simulink model "fuzzy_control_t2"  (R2017a)
settings: Solver=FixedStepAuto  StartTime=0.0  StopTime=10.0  FixedStep=0.0001  MaxStep=0.001  RelTol=1e-3
libraries: fuzblock x2
settings Model: Creator=Chaohua Zhao  LastModifiedBy=Chaohua Zhao

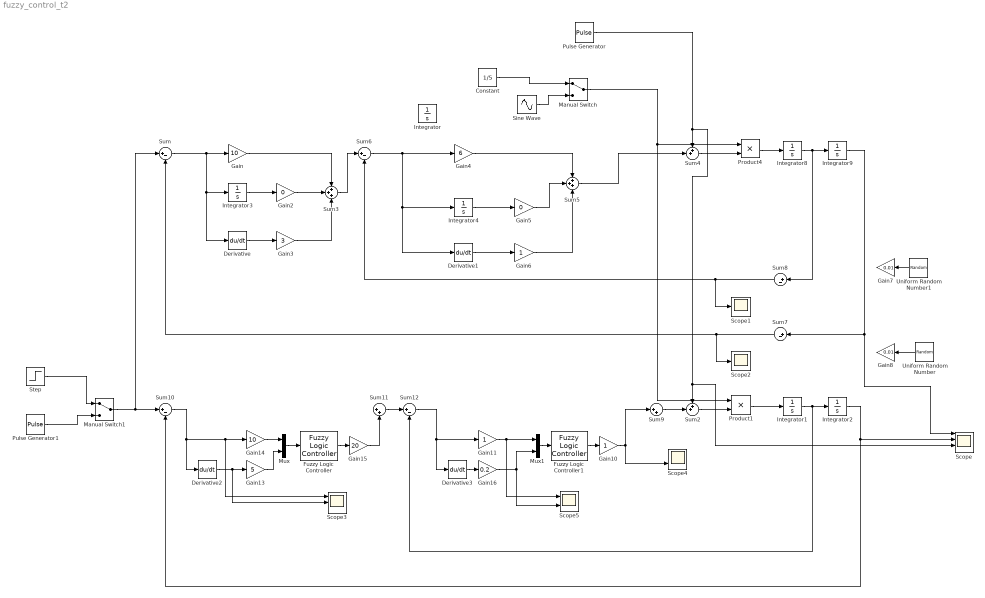
== system fuzzy_control_t2 ==
  Constant : Constant  Value=1/5
  Derivative{,1..3} (4 alike) : Derivative
  Fuzzy Logic Controller : fuzblock/Fuzzy Logic  Controller  fis=['fuzzy_sug_t2']
  Fuzzy Logic Controller1 : fuzblock/Fuzzy Logic  Controller  fis=['fuzzy_sug_t2']
  Gain : Gain  Gain=10
  Gain10 : Gain
  Gain11 : Gain
  Gain13 : Gain  Gain=5
  Gain14 : Gain  Gain=10
  Gain15 : Gain  Gain=20
  Gain16 : Gain  Gain=0.2
  Gain2 : Gain  Gain=0
  Gain3 : Gain  Gain=3
  Gain4 : Gain  Gain=6
  Gain5 : Gain  Gain=0
  Gain6 : Gain
  Gain7 : Gain  Gain=0.01
  Gain8 : Gain  Gain=0.01
  Integrator{,2..4,9} (5 alike) : Integrator
  Integrator1 : Integrator  LimitOutput=on  UpperSaturationLimit=100  LowerSaturationLimit=-100
  Integrator8 : Integrator  LimitOutput=on  UpperSaturationLimit=100  LowerSaturationLimit=-100
  Manual Switch : ManualSwitch
  Manual Switch1 : ManualSwitch
  Mux : Mux  Inputs=2
  Mux1 : Mux  Inputs=2
  Product1 : Product
  Product4 : Product
  Pulse Generator : DiscretePulseGenerator  PulseType=Time based  Amplitude=20  Period=3  PulseWidth=4  PhaseDelay=5
  Pulse Generator1 : DiscretePulseGenerator  PulseType=Time based  Period=15  PulseWidth=50
  Scope : Scope  NumInputPorts=4
  Scope1 : Scope
  Scope2 : Scope
  Scope3 : Scope  NumInputPorts=3
  Scope4 : Scope  NumInputPorts=2
  Scope5 : Scope  NumInputPorts=2
  Sine Wave : Sin  Amplitude=0.4  Bias=0.5  SampleTime=0
  Step : Step  Time=0  After=3  SampleTime=0
  Sum{,6..8,10,12} (6 alike) : Sum  Inputs=|+-
  Sum11 : Sum  Inputs=|++
  Sum2 : Sum  Inputs=++|
  Sum3 : Sum  Inputs=+++
  Sum4 : Sum  Inputs=++|
  Sum5 : Sum  Inputs=+++
  Sum9 : Sum  Inputs=|++
  Uniform Random Number : UniformRandomNumber  SampleTime=0.001
  Uniform Random Number1 : UniformRandomNumber  SampleTime=0.001
  wires:
  Integrator8/1 -> Integrator9/1, Sum8/1
  Sum4/1 -> Product4/2
  Product4/1 -> Integrator8/1
  Sine Wave/1 -> Manual Switch/2
  Constant/1 -> Manual Switch/1
  Product1/1 -> Integrator1/1
  Integrator1/1 -> Integrator2/1, Sum12/2
  Step/1 -> Manual Switch1/1
  Pulse Generator1/1 -> Manual Switch1/2
  Integrator9/1 -> Sum7/1, Scope/1
  Gain4/1 -> Sum5/1
  Derivative1/1 -> Gain6/1
  Integrator4/1 -> Gain5/1
  Sum6/1 -> Gain4/1, Derivative1/1, Integrator4/1
  Sum5/1 -> Sum4/2
  Sum3/1 -> Sum6/1
  Derivative/1 -> Gain3/1
  Integrator3/1 -> Gain2/1
  Gain/1 -> Sum3/1
  Sum/1 -> Derivative/1, Integrator3/1, Gain/1
  Gain3/1 -> Sum3/3
  Uniform Random Number/1 -> Gain8/1
  Uniform Random Number1/1 -> Gain7/1
  Sum8/1 -> Scope1/1, Sum6/2
  Sum7/1 -> Scope2/1, Sum/2
  Sum9/1 -> Sum2/2
  Mux/1 -> Fuzzy Logic Controller/1
  Gain13/1 -> Mux/2
  Gain14/1 -> Mux/1
  Sum10/1 -> Derivative2/1, Gain14/1, Scope3/1
  Fuzzy Logic Controller/1 -> Gain15/1
  Integrator2/1 -> Sum10/2, Scope/2
  Gain15/1 -> Sum11/2
  Derivative2/1 -> Gain13/1, Scope3/2
  Gain6/1 -> Sum5/3
  Sum12/1 -> Derivative3/1, Gain11/1
  Fuzzy Logic Controller1/1 -> Gain10/1
  Manual Switch1/1 -> Sum/1, Sum10/1
  Manual Switch/1 -> Product4/1, Product1/1
  Sum11/1 -> Sum12/1
  Gain5/1 -> Sum5/2
  Gain2/1 -> Sum3/2
  Gain10/1 -> Scope4/2, Sum9/1
  Mux1/1 -> Fuzzy Logic Controller1/1
  Derivative3/1 -> Gain16/1
  Gain11/1 -> Scope5/1, Mux1/1
  Gain16/1 -> Mux1/2, Scope5/2
  Sum2/1 -> Product1/2
  Pulse Generator/1 -> Scope/3, Sum2/1, Sum4/1
